simulink model "CSI_0313_SDC"  (R2019b)
settings: Solver=FixedStepDiscrete  StartTime=0.0  StopTime=Tstop  FixedStep=Tdelt  MaxStep=1e-4  RelTol=1e-3
values from neighbouring files (symbols this model uses):
  C = 12e-6    (= 1.2e-05)    [Inputparameter.m]
  Cdc = 4.76*10^-3    (= 0.00476)    [Inputparameter.m]
  Cemc = 1.5e-6    (= 1.5e-06)    [Inputparameter.m]
  enb = 0    [Run.m]
  fanalog = 7000    [Run.m]
  fTs = Update/18000    (= 0.000111111111111)    [Run.m]
  Ibase = 43*sqrt(2)    [Inputparameter.m]
  K120 = 0.0    (= 0)    [Run.m]
  K21 = 0.0    (= 0)    [Run.m]
  K5 = 0.0    (= 0)    [Run.m]
  K7 = 0.0    (= 0)    [Run.m]
  Kipll = 1.0    (= 1)    [Run.m]
  Klim = 1.03    [Run.m]
  Kpll = 20.0    (= 20)    [Run.m]
  Kpr = 0.9*Ibase/(Vbase)    [Run.m]
  Lgrid = 7.717e-4*10    (= 0.007717)    [Run.m]
  Lline = 60e-6    (= 6e-05)    [Inputparameter.m]
  Lpwm = 184.8e-6    (= 0.0001848)    [Inputparameter.m]
  mode = 1    [Run.m]
  Nsw = 18000/fbase    [Run.m]
  Qbpf = 1.0    (= 1)    [Run.m]
  Qpr = 1.0    (= 1)    [Run.m]
  Qs = 1    [Run.m]
  Rc = 10e-3    (= 0.01)    [Inputparameter.m]
  Remc = 1e-3    (= 0.001)    [Inputparameter.m]
  Rgrid = 2*pi*fbase*Lgrid/XR    [Run.m]
  Rline = 4.95e-3    (= 0.00495)    [Inputparameter.m]
  Rpre = 2.2    [Inputparameter.m]
  Rpwm = 6.2e-3    (= 0.0062)    [Inputparameter.m]
  Tdelt = (fTs)/(200*Update)    (= 2.77777777778e-07)    [Run.m]
  Tdt = 1.27e-6    (= 1.27e-06)    [Run.m]
  tstart = 0.2    [Run.m]
  Update = 2    [Run.m]
  Vbase = 400*sqrt(2/3)    [Inputparameter.m]
undefined symbols (not defined in the file or in its folder): sigbuilder_block
libraries: powerlib x54
(part 2 of 4)

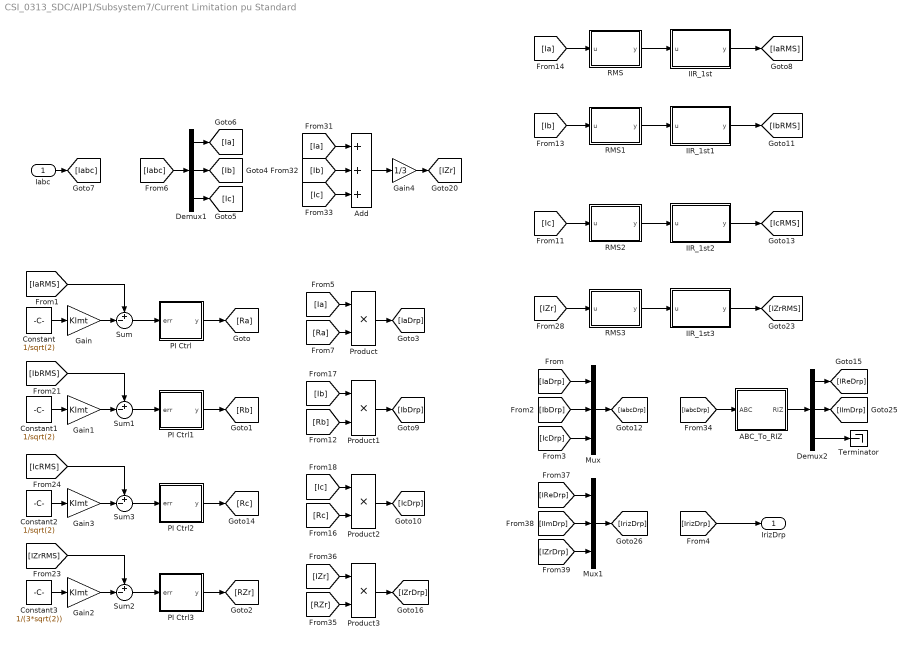
== system CSI_0313_SDC/AIP1/Subsystem7/Current Limitation pu Standard ==
  Iabc : Inport
  ABC_To_RIZ : MATLAB Function  TreatAsAtomicUnit=on
  Add : Sum  Inputs=+++
  Constant : Constant  Value=1/sqrt(2)
  Constant1 : Constant  Value=1/sqrt(2)
  Constant2 : Constant  Value=1/sqrt(2)
  Constant3 : Constant  Value=1/(3*sqrt(2))
  Demux1 : Demux  Outputs=3
  Demux2 : Demux  Outputs=3
  Gain{,1..3} (4 alike) : Gain  Gain=Klmt
  Gain4 : Gain  Gain=1/3
  IIR_1st : MATLAB Function  TreatAsAtomicUnit=on  mask{fc=100, fTs=fTs}
      mask prompts: fc "Cut-off frequency [Hz]"; fTs "Sample time [s]"
      mask help: 1st-order Low Pass Filter
  IIR_1st1 : MATLAB Function  TreatAsAtomicUnit=on  mask{fc=100, fTs=fTs}
      mask prompts: fc "Cut-off frequency [Hz]"; fTs "Sample time [s]"
      mask help: 1st-order Low Pass Filter
  IIR_1st2 : MATLAB Function  TreatAsAtomicUnit=on  mask{fc=100, fTs=fTs}
      mask prompts: fc "Cut-off frequency [Hz]"; fTs "Sample time [s]"
      mask help: 1st-order Low Pass Filter
  IIR_1st3 : MATLAB Function  TreatAsAtomicUnit=on  mask{fc=100, fTs=fTs}
      mask prompts: fc "Cut-off frequency [Hz]"; fTs "Sample time [s]"
      mask help: 1st-order Low Pass Filter
  Mux : Mux  Inputs=3
  Mux1 : Mux  Inputs=3
  PI Ctrl : MATLAB Function  TreatAsAtomicUnit=on  mask{fKP=0.005, fKI=100, fMinLmt=0, fMaxLmt=10, fTs=fTs}
      mask prompts: fKP "Proportional Gain"; fKI "Integral Coefficient"; fMinLmt "Minimum Limitation"; fMaxLmt "Maximum Limitation"; fTs "Sampling time [s]"
      mask help: Proportional Resonant Controller
  PI Ctrl1 : MATLAB Function  TreatAsAtomicUnit=on  mask{fKP=0.005, fKI=100, fMinLmt=0, fMaxLmt=10, fTs=fTs}
      mask prompts: fKP "Proportional Gain"; fKI "Integral Coefficient"; fMinLmt "Minimum Limitation"; fMaxLmt "Maximum Limitation"; fTs "Sampling time [s]"
      mask help: Proportional Resonant Controller
  PI Ctrl2 : MATLAB Function  TreatAsAtomicUnit=on  mask{fKP=0.005, fKI=100, fMinLmt=0, fMaxLmt=10, fTs=fTs}
      mask prompts: fKP "Proportional Gain"; fKI "Integral Coefficient"; fMinLmt "Minimum Limitation"; fMaxLmt "Maximum Limitation"; fTs "Sampling time [s]"
      mask help: Proportional Resonant Controller
  PI Ctrl3 : MATLAB Function  TreatAsAtomicUnit=on  mask{fKP=0.005, fKI=100, fMinLmt=0, fMaxLmt=10, fTs=fTs}
      mask prompts: fKP "Proportional Gain"; fKI "Integral Coefficient"; fMinLmt "Minimum Limitation"; fMaxLmt "Maximum Limitation"; fTs "Sampling time [s]"
      mask help: Proportional Resonant Controller
  Product{,1..3} (4 alike) : Product
  RMS : MATLAB Function  TreatAsAtomicUnit=on  mask{iNumAry=iRMSNum}
      mask prompts: iNumAry "RMS window points"
  RMS1 : MATLAB Function  TreatAsAtomicUnit=on  mask{iNumAry=iRMSNum}
      mask prompts: iNumAry "RMS window points"
  RMS2 : MATLAB Function  TreatAsAtomicUnit=on  mask{iNumAry=iRMSNum}
      mask prompts: iNumAry "RMS window points"
  RMS3 : MATLAB Function  TreatAsAtomicUnit=on  mask{iNumAry=iRMSNum}
      mask prompts: iNumAry "RMS window points"
  Sum{,1..3} (4 alike) : Sum  Inputs=+-|
  Terminator : Terminator
  IrizDrp : Outport
  wires:
  Demux2/3 -> Terminator/1
  Mux1/1 -> [IrizDrp]
  [IZrDrp] -> Mux1/3
  [IImDrp] -> Mux1/2
  [IReDrp] -> Mux1/1
  Demux2/2 -> [IImDrp]
  Demux2/1 -> [IReDrp]
  Product3/1 -> [IZrDrp]
  [RZr] -> Product3/2
  [IZr] -> Product3/1
  ABC_To_RIZ/1(RIZ) -> Demux2/1
  [IabcDrp] -> ABC_To_RIZ/1(ABC)
  Gain4/1 -> [IZr]
  [Ic] -> Add/3
  [Ib] -> Add/2
  [Ia] -> Add/1
  Add/1 -> Gain4/1
  Constant2/1 -> Gain3/1
  Sum3/1 -> PI Ctrl2/1(err)
  PI Ctrl2/1(y) -> [Rc]
  Gain3/1 -> Sum3/2
  [IcRMS] -> Sum3/1
  IIR_1st3/1(y) -> [IZrRMS]
  [IrizDrp] -> IrizDrp/1
  [IZr] -> RMS3/1(u)
  RMS3/1(y) -> IIR_1st3/1(u)
  Gain2/1 -> Sum2/2
  Constant3/1 -> Gain2/1
  Gain1/1 -> Sum1/2
  Constant1/1 -> Gain1/1
  Constant/1 -> Gain/1
  Gain/1 -> Sum/2
  IIR_1st2/1(y) -> [IcRMS]
  IIR_1st1/1(y) -> [IbRMS]
  IIR_1st/1(y) -> [IaRMS]
  RMS2/1(y) -> IIR_1st2/1(u)
  RMS1/1(y) -> IIR_1st1/1(u)
  RMS/1(y) -> IIR_1st/1(u)
  Sum2/1 -> PI Ctrl3/1(err)
  PI Ctrl3/1(y) -> [RZr]
  [IZrRMS] -> Sum2/1
  PI Ctrl1/1(y) -> [Rb]
  Sum1/1 -> PI Ctrl1/1(err)
  [IbRMS] -> Sum1/1
  Mux/1 -> [IabcDrp]
  Product2/1 -> [IcDrp]
  Product1/1 -> [IbDrp]
  Product/1 -> [IaDrp]
  [Rc] -> Product2/2
  [Ic] -> Product2/1
  [Rb] -> Product1/2
  [Ib] -> Product1/1
  [Ra] -> Product/2
  [Ia] -> Product/1
  Sum/1 -> PI Ctrl/1(err)
  [IcDrp] -> Mux/3
  [IbDrp] -> Mux/2
  [IaDrp] -> Mux/1
  PI Ctrl/1(y) -> [Ra]
  [IaRMS] -> Sum/1
  [Ib] -> RMS1/1(u)
  [Ic] -> RMS2/1(u)
  [Ia] -> RMS/1(u)
  Iabc/1 -> [Iabc]
  [Iabc] -> Demux1/1
  Demux1/1 -> [Ia]
  Demux1/3 -> [Ic]
  Demux1/2 -> [Ib]

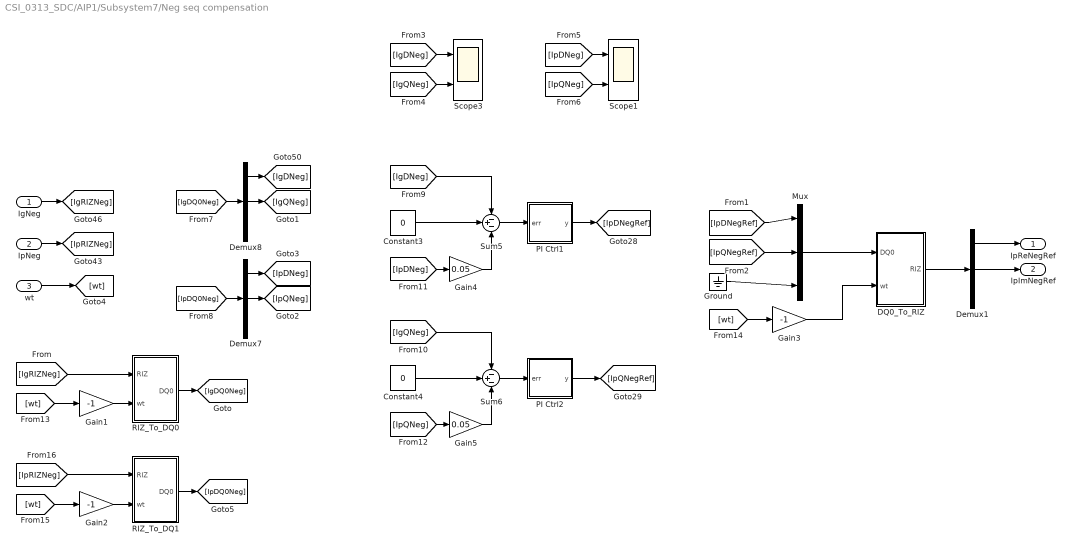
== system CSI_0313_SDC/AIP1/Subsystem7/Neg seq compensation ==
  IgNeg : Inport
  IpNeg : Inport  Port=2
  wt : Inport  Port=3
  Constant3 : Constant  Value=0  SampleTime=-1
  Constant4 : Constant  Value=0  SampleTime=-1
  DQ0_To_RIZ : MATLAB Function  TreatAsAtomicUnit=on  mask{iAxis=orient 90 degree behind A-axis}
      mask prompts: iAxis "Orient Axis Choice"
  Demux1 : Demux  Outputs=3
  Demux7 : Demux  Outputs=3
  Demux8 : Demux  Outputs=3
  Gain1 : Gain  Gain=-1
  Gain2 : Gain  Gain=-1
  Gain3 : Gain  Gain=-1
  Gain4 : Gain  Gain=0.05
  Gain5 : Gain  Gain=0.05
  Ground : Ground
  Mux : Mux  Inputs=3
  PI Ctrl1 : MATLAB Function  TreatAsAtomicUnit=on  mask{fKP=0.3, fKI=250, fMinLmt=-Ibase, fMaxLmt=Ibase, fTs=fTs}
      mask prompts: fKP "Proportional Gain"; fKI "Integral Coefficient"; fMinLmt "Minimum Limitation"; fMaxLmt "Maximum Limitation"; fTs "Sampling time [s]"
      mask help: Proportional Resonant Controller
  PI Ctrl2 : MATLAB Function  TreatAsAtomicUnit=on  mask{fKP=0.3, fKI=250, fMinLmt=-Ibase, fMaxLmt=Ibase, fTs=fTs}
      mask prompts: fKP "Proportional Gain"; fKI "Integral Coefficient"; fMinLmt "Minimum Limitation"; fMaxLmt "Maximum Limitation"; fTs "Sampling time [s]"
      mask help: Proportional Resonant Controller
  RIZ_To_DQ0 : MATLAB Function  TreatAsAtomicUnit=on  mask{iAxis=orient 90 degree behind A-axis}
      mask prompts: iAxis "Orient Axis Choice"
  RIZ_To_DQ1 : MATLAB Function  TreatAsAtomicUnit=on  mask{iAxis=orient 90 degree behind A-axis}
      mask prompts: iAxis "Orient Axis Choice"
  Scope1 : Scope  NumInputPorts=2
  Scope3 : Scope  NumInputPorts=2
  Sum5 : Sum  Inputs=-+-
  Sum6 : Sum  Inputs=-+-
  IpReNegRef : Outport  VectorParamsAs1DForOutWhenUnconnected=off
  IpImNegRef : Outport  Port=2  VectorParamsAs1DForOutWhenUnconnected=off
  wires:
  PI Ctrl1/1(y) -> [IpDNegRef]
  [IpQNeg] -> Gain5/1
  Demux8/2 -> [IgQNeg]
  Constant4/1 -> Sum6/2
  [IpDQ0Neg] -> Demux7/1
  Constant3/1 -> Sum5/2
  [IgDQ0Neg] -> Demux8/1
  Demux8/1 -> [IgDNeg]
  [IgDNeg] -> Sum5/1
  Demux7/2 -> [IpQNeg]
  [IpDNeg] -> Gain4/1
  [IgQNeg] -> Sum6/1
  Demux7/1 -> [IpDNeg]
  Sum5/1 -> PI Ctrl1/1(err)
  [IgDNeg] -> Scope3/1
  [IgQNeg] -> Scope3/2
  [IpDNeg] -> Scope1/1
  [IpQNeg] -> Scope1/2
  IgNeg/1 -> [IgRIZNeg]
  IpNeg/1 -> [IpRIZNeg]
  PI Ctrl2/1(y) -> [IpQNegRef]
  Sum6/1 -> PI Ctrl2/1(err)
  [IgRIZNeg] -> RIZ_To_DQ0/1(RIZ)
  wt/1 -> [wt]
  [wt] -> Gain1/1
  Gain1/1 -> RIZ_To_DQ0/2(wt)
  RIZ_To_DQ0/1(DQ0) -> [IgDQ0Neg]
  RIZ_To_DQ1/1(DQ0) -> [IpDQ0Neg]
  Gain2/1 -> RIZ_To_DQ1/2(wt)
  [wt] -> Gain2/1
  [IpRIZNeg] -> RIZ_To_DQ1/1(RIZ)
  [IpDNegRef] -> Mux/1
  [IpQNegRef] -> Mux/2
  Ground/1 -> Mux/3
  Mux/1 -> DQ0_To_RIZ/1(DQ0)
  [wt] -> Gain3/1
  Gain3/1 -> DQ0_To_RIZ/2(wt)
  DQ0_To_RIZ/1(RIZ) -> Demux1/1
  Demux1/1 -> IpReNegRef/1
  Demux1/2 -> IpImNegRef/1
  Gain4/1 -> Sum5/3
  Gain5/1 -> Sum6/3

== system CSI_0313_SDC/AIP1/Subsystem7/PLL ==
  Vabc : Inport
  ABC_To_RIZ : MATLAB Function  TreatAsAtomicUnit=on
  Constant : Constant  Value=2*pi*fFqBase  SampleTime=-1
  Constant1 : Constant  Value=2*pi
  Delay1 : Delay  DelayLength=1
  Delay2 : Delay  DelayLength=1
  Demux3 : Demux  Outputs=3
  Gain : Gain  Gain=1/(2*pi)
  Integral : MATLAB Function  TreatAsAtomicUnit=on  mask{fGain=1.0, fTs=fTs}
      mask prompts: fGain "Gain Value"; fTs "Sampling time [s]"
      mask help: Proportional Resonant Controller
  Math Function : Math  Operator=mod  SaturateOnIntegerOverflow=on
  PI Ctrl : MATLAB Function  TreatAsAtomicUnit=on  mask{fKP=fKPPLL, fKI=fKIPLL, fMinLmt=fDltMin, fMaxLmt=fDltMax, fTs=fTs}
      mask prompts: fKP "Proportional Gain"; fKI "Integral Coefficient"; fMinLmt "Minimum Limitation"; fMaxLmt "Maximum Limitation"; fTs "Sampling time [s]"
      mask help: Proportional Resonant Controller
  "Pos&Neg seq extract in subsystem " : Subsystem  mask{fQ=1.0, fTs=fTs}
      mask prompts: fQ "Quality Factor"; fTs "Sample Time"
  RIZ_To_DQ0 : MATLAB Function  TreatAsAtomicUnit=on  mask{iAxis=orient in A-axis}
      mask prompts: iAxis "Orient Axis Choice"
  Scope : Scope
  Sum : Sum  Inputs=++|
  Terminator : Terminator
  Terminator1 : Terminator
  f : Outport
  wt : Outport  Port=2
  VdPos : Outport  Port=3
  wires:
  Delay1/1 -> "Pos&Neg seq extract in subsystem "/2(ffc)
  "Pos&Neg seq extract in subsystem "/3(chk) -> [chk]
  [VdPos] -> VdPos/1
  [f] -> Delay1/1
  Demux3/3 -> Terminator1/1
  "Pos&Neg seq extract in subsystem "/2(RizNeg) -> Terminator/1
  "Pos&Neg seq extract in subsystem "/1(RizPos) -> [VrizPos]
  [Vriz] -> "Pos&Neg seq extract in subsystem "/1(RIZ)
  RIZ_To_DQ0/1(DQ0) -> Scope/1, [Vdq0Pos]
  [w] -> Gain/1
  [w] -> Integral/1(u)
  Gain/1 -> [f]
  Demux3/2 -> [VqPos]
  Demux3/1 -> [VdPos]
  [Vdq0Pos] -> Demux3/1
  PI Ctrl/1(y) -> Sum/2
  Sum/1 -> [w]
  [VrizPos] -> RIZ_To_DQ0/1(RIZ)
  Constant/1 -> Sum/1
  Vabc/1 -> [Vabc]
  Integral/1(y) -> Math Function/1
  Constant1/1 -> Math Function/2
  Math Function/1 -> [wt]
  [VqPos] -> PI Ctrl/1(err)
  [f] -> f/1
  [wt] -> Delay2/1
  Delay2/1 -> RIZ_To_DQ0/2(wt)
  [Vabc] -> ABC_To_RIZ/1(ABC)
  ABC_To_RIZ/1(RIZ) -> [Vriz]
  [wt] -> wt/1

== system CSI_0313_SDC/AIP1/Subsystem7/PR CSI Loop ==
  IrizRef : Inport
  Iriz : Inport  Port=2
  IrizDrp : Inport  Port=3
  fPLL : Inport  Port=4
  Demux1 : Demux  Outputs=3
  Demux2 : Demux  Outputs=3
  Demux3 : Demux  Outputs=3
  Mux3 : Mux  Inputs=3
  PR Ctrl : MATLAB Function  TreatAsAtomicUnit=on  mask{fP=fKP, fQ=fKQ, fTs=fTs}
      mask prompts: fP "Proportional Gain"; fQ "Quality Factor"; fTs "Sampling time [s]"
      mask help: Proportional Resonant Controller
  PR Ctrl1 : MATLAB Function  TreatAsAtomicUnit=on  mask{fP=fKP, fQ=fKQ, fTs=fTs}
      mask prompts: fP "Proportional Gain"; fQ "Quality Factor"; fTs "Sampling time [s]"
      mask help: Proportional Resonant Controller
  PR Ctrl2 : MATLAB Function  TreatAsAtomicUnit=on  mask{fP=fKP*mode, fQ=fKQ, fTs=fTs}
      mask prompts: fP "Proportional Gain"; fQ "Quality Factor"; fTs "Sampling time [s]"
      mask help: Proportional Resonant Controller
  RIZ_To_ABC : MATLAB Function  TreatAsAtomicUnit=on
  Sum : Sum  Inputs=-+-
  Sum1 : Sum  Inputs=-+-
  Sum2 : Sum  Inputs=-+-
  VabcFB : Outport
  wires:
  Sum2/1 -> PR Ctrl2/1(err)
  Sum1/1 -> PR Ctrl1/1(err)
  Sum/1 -> PR Ctrl/1(err)
  [VabcFB] -> VabcFB/1
  fPLL/1 -> [fPLL]
  IrizDrp/1 -> [IrizDrp]
  [IrizDrp] -> Demux2/1
  Demux2/3 -> [IZrDrp]
  Demux2/1 -> [IReDrp]
  Demux2/2 -> [IImDrp]
  Demux1/2 -> [IImRef]
  [IrizRef] -> Demux1/1
  Demux1/1 -> [IReRef]
  Demux1/3 -> [IZrRef]
  IrizRef/1 -> [IrizRef]
  Iriz/1 -> [Iriz]
  Demux3/3 -> [IZr]
  Demux3/1 -> [IRe]
  Demux3/2 -> [IIm]
  [Iriz] -> Demux3/1
  PR Ctrl2/1(y) -> [VZrFB]
  [IImDrp] -> Sum1/3
  [IZr] -> Sum2/1
  Mux3/1 -> RIZ_To_ABC/1(RIZ)
  [fPLL] -> PR Ctrl1/2(ffc)
  RIZ_To_ABC/1(ABC) -> [VabcFB]
  [IReDrp] -> Sum/3
  [fPLL] -> PR Ctrl/2(ffc)
  [IIm] -> Sum1/1
  [fPLL] -> PR Ctrl2/2(ffc)
  [IImRef] -> Sum1/2
  [VReFB] -> Mux3/1
  [VZrFB] -> Mux3/3
  [IRe] -> Sum/1
  PR Ctrl1/1(y) -> [VImFB]
  PR Ctrl/1(y) -> [VReFB]
  [IZrRef] -> Sum2/2
  [IZrDrp] -> Sum2/3
  [IReRef] -> Sum/2
  [VImFB] -> Mux3/2

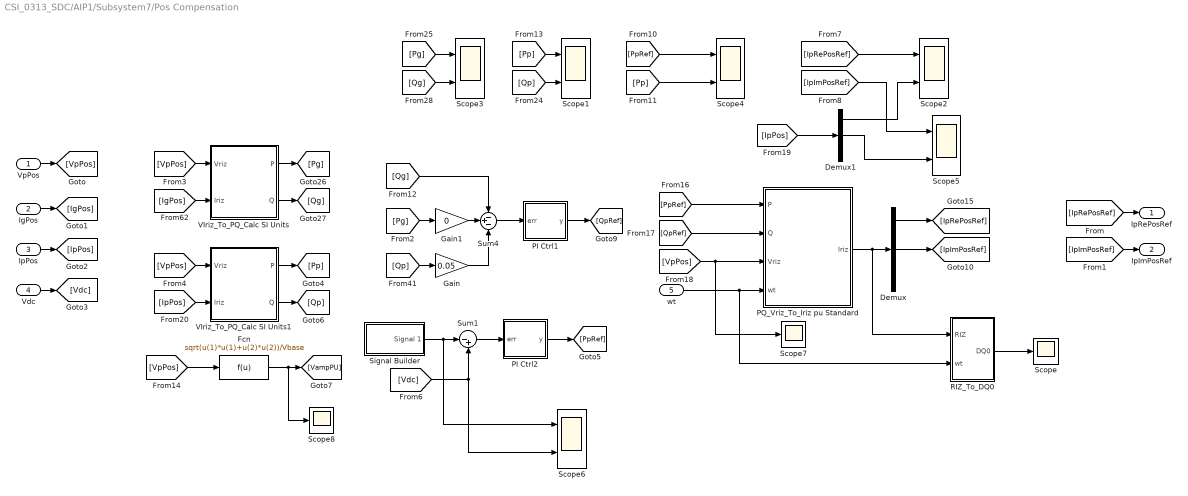
== system CSI_0313_SDC/AIP1/Subsystem7/Pos Compensation ==
  VpPos : Inport
  IgPos : Inport  Port=2
  IpPos : Inport  Port=3
  Vdc : Inport  Port=4
  wt : Inport  Port=5
  Demux : Demux  Outputs=3
  Demux1 : Demux  Outputs=3
  Fcn : Fcn  Expr=sqrt(u(1)*u(1)+u(2)*u(2))/Vbase
  Gain : Gain  Gain=0.05
  Gain1 : Gain  Gain=0
  PI Ctrl1 : MATLAB Function  TreatAsAtomicUnit=on  mask{fKP=0.3, fKI=200, fMinLmt=-30, fMaxLmt=30, fTs=fTs}
      mask prompts: fKP "Proportional Gain"; fKI "Integral Coefficient"; fMinLmt "Minimum Limitation"; fMaxLmt "Maximum Limitation"; fTs "Sampling time [s]"
      mask help: Proportional Resonant Controller
  PI Ctrl2 : MATLAB Function  TreatAsAtomicUnit=on  mask{fKP=0.05, fKI=0, fMinLmt=-30, fMaxLmt=30, fTs=fTs}
      mask prompts: fKP "Proportional Gain"; fKI "Integral Coefficient"; fMinLmt "Minimum Limitation"; fMaxLmt "Maximum Limitation"; fTs "Sampling time [s]"
      mask help: Proportional Resonant Controller
  PQ_Vriz_To_Iriz pu Standard : MATLAB Function  TreatAsAtomicUnit=on  mask{Ibase=Ibase}
      mask prompts: Ibase "Current base"
  RIZ_To_DQ0 : MATLAB Function  TreatAsAtomicUnit=on  mask{iAxis=orient 90 degree behind A-axis}
      mask prompts: iAxis "Orient Axis Choice"
  Scope : Scope
  Scope{1..6} (6 alike) : Scope  NumInputPorts=2
  Scope7 : Scope
  Scope8 : Scope
  Signal Builder : Subsystem  Tag=STV Subsys  LoadFcn=sigbuilder_block('load');  StartFcn=sigbuilder_block('start');  StopFcn=sigbuilder_block('stop');  ClipboardFcn=sigbuilder_block('clipboard');  mask(Sigbuilder block){tuvar=[0:10]}
      mask help: Simulink:masks:SigbuilderBlock_MD
      mask init:
      | if ~strcmp(get_param(bdroot(gcbh),'SimulationStatus'),'stopped') tuvar = sigbuilder_block('maskInit'); end
      settings: CopyFcn=sigbuilder_block('copy');  DeleteFcn=sigbuilder_block('delete');  ModelCloseFcn=sigbuilder_block('modelClose');  PreSaveFcn=sigbuilder_block('preSave');  PauseFcn=sigbuilder_block('pause');  ContinueFcn=sigbuilder_block('continue');  NameChangeFcn=sigbuilder_block('namechange');  OpenFcn=sigbuilder_block('open',[403.2 79.8 550.8 400.2 ]);  CloseFcn=sigbuilder_block('close');
      mask Display: plot(0, 0, 100, 100,[2, 2, 32, 32, 2], [68, 8, 8, 68, 68],[32, 2], [38, 38], [32, 19, 2],[53, 60, 44], [32, 17, 17, 2],[16, 16, 31, 31]);txt = getActiveGroup(gcbh);text(2, 100, txt,'verticalAlignment', 'top');
  Sum1 : Sum  Inputs=|-+
  Sum4 : Sum  Inputs=-+-
  VIriz_To_PQ_Calc SI Units : MATLAB Function  TreatAsAtomicUnit=on
  VIriz_To_PQ_Calc SI Units1 : MATLAB Function  TreatAsAtomicUnit=on
  IpRePosRef : Outport  VectorParamsAs1DForOutWhenUnconnected=off
  IpImPosRef : Outport  Port=2  VectorParamsAs1DForOutWhenUnconnected=off
  wires:
  [VpPos] -> VIriz_To_PQ_Calc SI Units/1(Vriz)
  VIriz_To_PQ_Calc SI Units/2(Q) -> [Qg]
  [IpPos] -> VIriz_To_PQ_Calc SI Units1/2(Iriz)
  VIriz_To_PQ_Calc SI Units1/2(Q) -> [Qp]
  [IgPos] -> VIriz_To_PQ_Calc SI Units/2(Iriz)
  [Qp] -> Gain/1
  VIriz_To_PQ_Calc SI Units1/1(P) -> [Pp]
  Sum4/1 -> PI Ctrl1/1(err)
  [VpPos] -> VIriz_To_PQ_Calc SI Units1/1(Vriz)
  VIriz_To_PQ_Calc SI Units/1(P) -> [Pg]
  PI Ctrl1/1(y) -> [QpRef]
  Gain/1 -> Sum4/3
  [Qg] -> Scope3/2
  [Qg] -> Sum4/1
  [Pg] -> Scope3/1
  Demux/1 -> [IpRePosRef]
  [Pp] -> Scope1/1
  Demux/2 -> [IpImPosRef]
  VpPos/1 -> [VpPos]
  IgPos/1 -> [IgPos]
  IpPos/1 -> [IpPos]
  [IpRePosRef] -> IpRePosRef/1
  [IpImPosRef] -> IpImPosRef/1
  [Qp] -> Scope1/2
  [Pg] -> Gain1/1
  Gain1/1 -> Sum4/2
  Vdc/1 -> [Vdc]
  Sum1/1 -> PI Ctrl2/1(err)
  PI Ctrl2/1(y) -> [PpRef]
  [PpRef] -> Scope4/1
  [Pp] -> Scope4/2
  wt/1 -> RIZ_To_DQ0/2(wt), PQ_Vriz_To_Iriz pu Standard/4(wt)
  [VpPos] -> Fcn/1
  Fcn/1 -> Scope8/1, [VampPU]
  [PpRef] -> PQ_Vriz_To_Iriz pu Standard/1(P)
  [QpRef] -> PQ_Vriz_To_Iriz pu Standard/2(Q)
  [IpPos] -> Demux1/1
  [IpRePosRef] -> Scope2/1
  Demux1/1 -> Scope2/2
  [IpImPosRef] -> Scope5/1
  Demux1/2 -> Scope5/2
  PQ_Vriz_To_Iriz pu Standard/1(Iriz) -> RIZ_To_DQ0/1(RIZ), Demux/1
  [Vdc] -> Scope6/2, Sum1/2
  Signal Builder/1(Signal 1) -> Scope6/1, Sum1/1
  RIZ_To_DQ0/1(DQ0) -> Scope/1
  [VpPos] -> PQ_Vriz_To_Iriz pu Standard/3(Vriz), Scope7/1

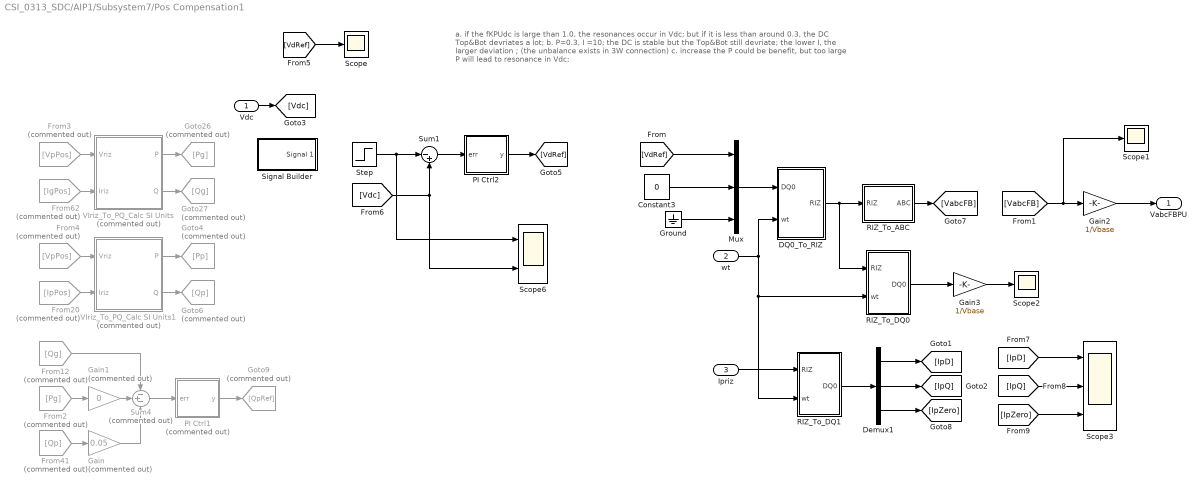
== system CSI_0313_SDC/AIP1/Subsystem7/Pos Compensation1 ==
  note: a. if the fKPUdc is large than 1.0, the resonances occur in Vdc; but if it is less than around 0.3, the DC Top&Bot devriates a lot;
      | b. P=0.3, I =10; the DC is stable but the Top&Bot still devriate; the lower I, the larger deviation；(the unbalance exists in 3W connection)
      | c. increase the P could be benefit, but too large P will lead to resonance in Vdc;
  Vdc : Inport
  wt : Inport  Port=2
  Ipriz : Inport  Port=3
  Constant3 : Constant  Value=0  SampleTime=-1
  DQ0_To_RIZ : MATLAB Function  TreatAsAtomicUnit=on  mask{iAxis=orient in A-axis}
      mask prompts: iAxis "Orient Axis Choice"
  Demux1 : Demux  Outputs=3
  From12 : From  Commented=on  GotoTag=Qg
  From2 : From  Commented=on  GotoTag=Pg
  From20 : From  Commented=on  GotoTag=IpPos
  From3 : From  Commented=on  GotoTag=VpPos
  From4 : From  Commented=on  GotoTag=VpPos
  From41 : From  Commented=on  GotoTag=Qp
  From62 : From  Commented=on  GotoTag=IgPos
  Gain : Gain  Commented=on  Gain=0.05
  Gain1 : Gain  Commented=on  Gain=0
  Gain2 : Gain  Gain=1/Vbase
  Gain3 : Gain  Gain=1/Vbase
  Goto26 : Goto  Commented=on  GotoTag=Pg
  Goto27 : Goto  Commented=on  GotoTag=Qg
  Goto4 : Goto  Commented=on  GotoTag=Pp
  Goto6 : Goto  Commented=on  GotoTag=Qp
  Goto9 : Goto  Commented=on  GotoTag=QpRef
  Ground : Ground
  Mux : Mux  Inputs=3
  PI Ctrl1 : MATLAB Function  Commented=on  TreatAsAtomicUnit=on  mask{fKP=0.3, fKI=200, fMinLmt=-30, fMaxLmt=30, fTs=fTs}
      mask prompts: fKP "Proportional Gain"; fKI "Integral Coefficient"; fMinLmt "Minimum Limitation"; fMaxLmt "Maximum Limitation"; fTs "Sampling time [s]"
      mask help: Proportional Resonant Controller
  PI Ctrl2 : MATLAB Function  TreatAsAtomicUnit=on  mask{fKP=0.4, fKI=6, fMinLmt=-0.3*Vbase, fMaxLmt=0.3*Vbase, fTs=fTs}
      mask prompts: fKP "Proportional Gain"; fKI "Integral Coefficient"; fMinLmt "Minimum Limitation"; fMaxLmt "Maximum Limitation"; fTs "Sampling time [s]"
      mask help: Proportional Resonant Controller
  RIZ_To_ABC : MATLAB Function  TreatAsAtomicUnit=on
  RIZ_To_DQ0 : MATLAB Function  TreatAsAtomicUnit=on  mask{iAxis=orient in A-axis}
      mask prompts: iAxis "Orient Axis Choice"
  RIZ_To_DQ1 : MATLAB Function  TreatAsAtomicUnit=on  mask{iAxis=orient in A-axis}
      mask prompts: iAxis "Orient Axis Choice"
  Scope : Scope
  Scope1 : Scope
  Scope2 : Scope
  Scope3 : Scope  NumInputPorts=3
  Scope6 : Scope  NumInputPorts=2
  Signal Builder : Subsystem  Tag=STV Subsys  LoadFcn=sigbuilder_block('load');  StartFcn=sigbuilder_block('start');  StopFcn=sigbuilder_block('stop');  ClipboardFcn=sigbuilder_block('clipboard');  mask(Sigbuilder block){tuvar=[0:10]}
      mask help: Simulink:masks:SigbuilderBlock_MD
      mask init:
      | if ~strcmp(get_param(bdroot(gcbh),'SimulationStatus'),'stopped') tuvar = sigbuilder_block('maskInit'); end
      settings: CopyFcn=sigbuilder_block('copy');  DeleteFcn=sigbuilder_block('delete');  ModelCloseFcn=sigbuilder_block('modelClose');  PreSaveFcn=sigbuilder_block('preSave');  PauseFcn=sigbuilder_block('pause');  ContinueFcn=sigbuilder_block('continue');  NameChangeFcn=sigbuilder_block('namechange');  OpenFcn=sigbuilder_block('open',[403.2 79.8 550.8 400.2 ]);  CloseFcn=sigbuilder_block('close');
      mask Display: plot(0, 0, 100, 100,[2, 2, 32, 32, 2], [68, 8, 8, 68, 68],[32, 2], [38, 38], [32, 19, 2],[53, 60, 44], [32, 17, 17, 2],[16, 16, 31, 31]);txt = getActiveGroup(gcbh);text(2, 100, txt,'verticalAlignment', 'top');
  Step : Step  Time=0.5  Before=650  After=700
  Sum1 : Sum  Inputs=|-+
  Sum4 : Sum  Commented=on  Inputs=-+-
  VIriz_To_PQ_Calc SI Units : MATLAB Function  Commented=on  TreatAsAtomicUnit=on
  VIriz_To_PQ_Calc SI Units1 : MATLAB Function  Commented=on  TreatAsAtomicUnit=on
  VabcFBPU : Outport  VectorParamsAs1DForOutWhenUnconnected=off
  wires:
  [Vdc] -> Sum1/2, Scope6/2
  PI Ctrl2/1(y) -> [VdRef]
  Sum1/1 -> PI Ctrl2/1(err)
  Vdc/1 -> [Vdc]
  Gain1/1 -> Sum4/2
  From2/1 -> Gain1/1
  [VabcFB] -> Scope1/1, Gain2/1
  [VdRef] -> Scope/1
  From12/1 -> Sum4/1
  Gain/1 -> Sum4/3
  PI Ctrl1/1(y) -> Goto9/1
  VIriz_To_PQ_Calc SI Units/1(P) -> Goto26/1
  From4/1 -> VIriz_To_PQ_Calc SI Units1/1(Vriz)
  Sum4/1 -> PI Ctrl1/1(err)
  VIriz_To_PQ_Calc SI Units1/1(P) -> Goto4/1
  From41/1 -> Gain/1
  From62/1 -> VIriz_To_PQ_Calc SI Units/2(Iriz)
  VIriz_To_PQ_Calc SI Units1/2(Q) -> Goto6/1
  From20/1 -> VIriz_To_PQ_Calc SI Units1/2(Iriz)
  VIriz_To_PQ_Calc SI Units/2(Q) -> Goto27/1
  From3/1 -> VIriz_To_PQ_Calc SI Units/1(Vriz)
  Ground/1 -> Mux/3
  Mux/1 -> DQ0_To_RIZ/1(DQ0)
  wt/1 -> RIZ_To_DQ0/2(wt), RIZ_To_DQ1/2(wt), DQ0_To_RIZ/2(wt)
  RIZ_To_ABC/1(ABC) -> [VabcFB]
  DQ0_To_RIZ/1(RIZ) -> RIZ_To_DQ0/1(RIZ), RIZ_To_ABC/1(RIZ)
  Gain2/1 -> VabcFBPU/1
  RIZ_To_DQ0/1(DQ0) -> Gain3/1
  Gain3/1 -> Scope2/1
  Step/1 -> Scope6/1, Sum1/1
  [VdRef] -> Mux/1
  Ipriz/1 -> RIZ_To_DQ1/1(RIZ)
  RIZ_To_DQ1/1(DQ0) -> Demux1/1
  Demux1/1 -> [IpD]
  Demux1/2 -> [IpQ]
  Constant3/1 -> Mux/2
  [IpD] -> Scope3/1
  [IpQ] -> Scope3/2
  Demux1/3 -> [IpZero]
  [IpZero] -> Scope3/3

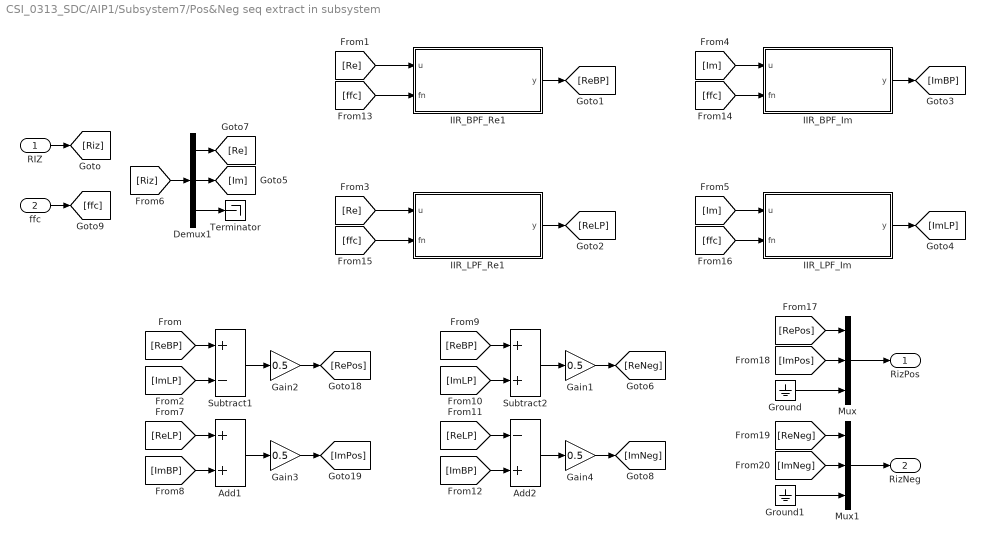
== system CSI_0313_SDC/AIP1/Subsystem7/Pos&Neg seq extract in subsystem  ==
  RIZ : Inport
  ffc : Inport  Port=2
  Add1 : Sum
  Add2 : Sum  Inputs=-+
  Demux1 : Demux  Outputs=3
  Gain{1..4} (4 alike) : Gain  Gain=0.5
  Ground : Ground
  Ground1 : Ground
  IIR_BPF_Im : MATLAB Function  TreatAsAtomicUnit=on  mask{fQ=fQ, fTs=fTs, iMode=IIR2 used as BPF in SOGI}
      mask prompts: fQ "Quality factor"; fTs "Sample time [s]"; iMode "Modes of 2nd-order transfer function"
  IIR_BPF_Re1 : MATLAB Function  TreatAsAtomicUnit=on  mask{fQ=fQ, fTs=fTs, iMode=IIR2 used as BPF in SOGI}
      mask prompts: fQ "Quality factor"; fTs "Sample time [s]"; iMode "Modes of 2nd-order transfer function"
  IIR_LPF_Im : MATLAB Function  TreatAsAtomicUnit=on  mask{fQ=fQ, fTs=fTs, iMode=IIR2 used as LPF in SOGI}
      mask prompts: fQ "Quality factor"; fTs "Sample time [s]"; iMode "Modes of 2nd-order transfer function"
  IIR_LPF_Re1 : MATLAB Function  TreatAsAtomicUnit=on  mask{fQ=fQ, fTs=fTs, iMode=IIR2 used as LPF in SOGI}
      mask prompts: fQ "Quality factor"; fTs "Sample time [s]"; iMode "Modes of 2nd-order transfer function"
  Mux : Mux  Inputs=3
  Mux1 : Mux  Inputs=3
  Subtract1 : Sum  Inputs=+-
  Subtract2 : Sum
  Terminator : Terminator
  RizPos : Outport
  RizNeg : Outport  Port=2
  wires:
  [ImBP] -> Add2/2
  [ffc] -> IIR_BPF_Im/2(fn)
  Add1/1 -> Gain3/1
  Demux1/1 -> [Re]
  RIZ/1 -> [Riz]
  Ground1/1 -> Mux1/3
  Add2/1 -> Gain4/1
  [ImLP] -> Subtract1/2
  [ReLP] -> Add1/1
  [ReBP] -> Subtract2/1
  [ImBP] -> Add1/2
  Gain1/1 -> [ReNeg]
  IIR_LPF_Re1/1(y) -> [ReLP]
  [Re] -> IIR_BPF_Re1/1(u)
  [RePos] -> Mux/1
  [ReBP] -> Subtract1/1
  Mux/1 -> RizPos/1
  [ffc] -> IIR_BPF_Re1/2(fn)
  Mux1/1 -> RizNeg/1
  IIR_BPF_Im/1(y) -> [ImBP]
  [Im] -> IIR_BPF_Im/1(u)
  Demux1/3 -> Terminator/1
  IIR_BPF_Re1/1(y) -> [ReBP]
  Gain3/1 -> [ImPos]
  IIR_LPF_Im/1(y) -> [ImLP]
  [ImNeg] -> Mux1/2
  [Im] -> IIR_LPF_Im/1(u)
  [ffc] -> IIR_LPF_Im/2(fn)
  [ImLP] -> Subtract2/2
  Demux1/2 -> [Im]
  Subtract1/1 -> Gain2/1
  [Re] -> IIR_LPF_Re1/1(u)
  [ffc] -> IIR_LPF_Re1/2(fn)
  [Riz] -> Demux1/1
  Ground/1 -> Mux/3
  [ReNeg] -> Mux1/1
  Gain4/1 -> [ImNeg]
  Subtract2/1 -> Gain1/1
  Gain2/1 -> [RePos]
  [ReLP] -> Add2/1
  ffc/1 -> [ffc]
  [ImPos] -> Mux/2

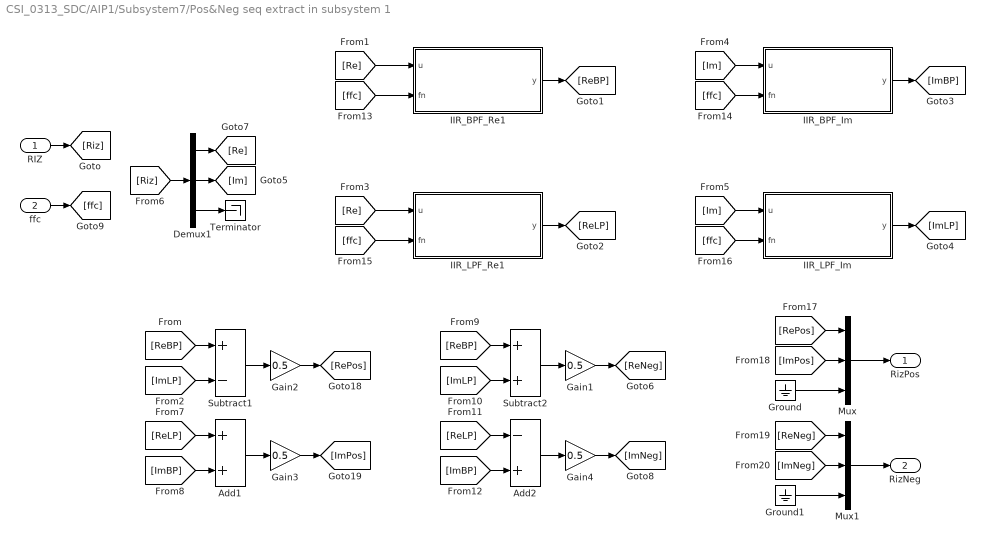
== system CSI_0313_SDC/AIP1/Subsystem7/Pos&Neg seq extract in subsystem 1 ==
  RIZ : Inport
  ffc : Inport  Port=2
  Add1 : Sum
  Add2 : Sum  Inputs=-+
  Demux1 : Demux  Outputs=3
  Gain{1..4} (4 alike) : Gain  Gain=0.5
  Ground : Ground
  Ground1 : Ground
  IIR_BPF_Im : MATLAB Function  TreatAsAtomicUnit=on  mask{fQ=fQ, fTs=fTs, iMode=IIR2 used as BPF in SOGI}
      mask prompts: fQ "Quality factor"; fTs "Sample time [s]"; iMode "Modes of 2nd-order transfer function"
  IIR_BPF_Re1 : MATLAB Function  TreatAsAtomicUnit=on  mask{fQ=fQ, fTs=fTs, iMode=IIR2 used as BPF in SOGI}
      mask prompts: fQ "Quality factor"; fTs "Sample time [s]"; iMode "Modes of 2nd-order transfer function"
  IIR_LPF_Im : MATLAB Function  TreatAsAtomicUnit=on  mask{fQ=fQ, fTs=fTs, iMode=IIR2 used as LPF in SOGI}
      mask prompts: fQ "Quality factor"; fTs "Sample time [s]"; iMode "Modes of 2nd-order transfer function"
  IIR_LPF_Re1 : MATLAB Function  TreatAsAtomicUnit=on  mask{fQ=fQ, fTs=fTs, iMode=IIR2 used as LPF in SOGI}
      mask prompts: fQ "Quality factor"; fTs "Sample time [s]"; iMode "Modes of 2nd-order transfer function"
  Mux : Mux  Inputs=3
  Mux1 : Mux  Inputs=3
  Subtract1 : Sum  Inputs=+-
  Subtract2 : Sum
  Terminator : Terminator
  RizPos : Outport
  RizNeg : Outport  Port=2
  wires:
  [ImPos] -> Mux/2
  ffc/1 -> [ffc]
  [ReLP] -> Add2/1
  Gain2/1 -> [RePos]
  Subtract2/1 -> Gain1/1
  Gain4/1 -> [ImNeg]
  [ReNeg] -> Mux1/1
  Ground/1 -> Mux/3
  [Riz] -> Demux1/1
  [ffc] -> IIR_LPF_Re1/2(fn)
  [Re] -> IIR_LPF_Re1/1(u)
  Subtract1/1 -> Gain2/1
  Demux1/2 -> [Im]
  [ImLP] -> Subtract2/2
  [ffc] -> IIR_LPF_Im/2(fn)
  [Im] -> IIR_LPF_Im/1(u)
  [ImNeg] -> Mux1/2
  IIR_LPF_Im/1(y) -> [ImLP]
  Gain3/1 -> [ImPos]
  IIR_BPF_Re1/1(y) -> [ReBP]
  Demux1/3 -> Terminator/1
  [Im] -> IIR_BPF_Im/1(u)
  IIR_BPF_Im/1(y) -> [ImBP]
  Mux1/1 -> RizNeg/1
  [ffc] -> IIR_BPF_Re1/2(fn)
  Mux/1 -> RizPos/1
  [ReBP] -> Subtract1/1
  [RePos] -> Mux/1
  [Re] -> IIR_BPF_Re1/1(u)
  IIR_LPF_Re1/1(y) -> [ReLP]
  Gain1/1 -> [ReNeg]
  [ImBP] -> Add1/2
  [ReBP] -> Subtract2/1
  [ReLP] -> Add1/1
  [ImLP] -> Subtract1/2
  Add2/1 -> Gain4/1
  Ground1/1 -> Mux1/3
  RIZ/1 -> [Riz]
  Demux1/1 -> [Re]
  Add1/1 -> Gain3/1
  [ffc] -> IIR_BPF_Im/2(fn)
  [ImBP] -> Add2/2

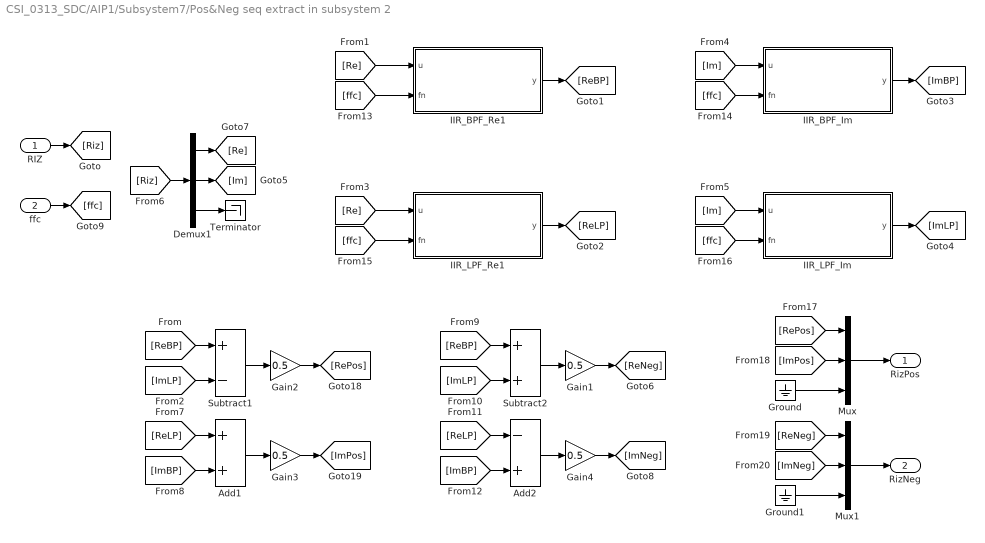
== system CSI_0313_SDC/AIP1/Subsystem7/Pos&Neg seq extract in subsystem 2 ==
  RIZ : Inport
  ffc : Inport  Port=2
  Add1 : Sum
  Add2 : Sum  Inputs=-+
  Demux1 : Demux  Outputs=3
  Gain{1..4} (4 alike) : Gain  Gain=0.5
  Ground : Ground
  Ground1 : Ground
  IIR_BPF_Im : MATLAB Function  TreatAsAtomicUnit=on  mask{fQ=fQ, fTs=fTs, iMode=IIR2 used as BPF in SOGI}
      mask prompts: fQ "Quality factor"; fTs "Sample time [s]"; iMode "Modes of 2nd-order transfer function"
  IIR_BPF_Re1 : MATLAB Function  TreatAsAtomicUnit=on  mask{fQ=fQ, fTs=fTs, iMode=IIR2 used as BPF in SOGI}
      mask prompts: fQ "Quality factor"; fTs "Sample time [s]"; iMode "Modes of 2nd-order transfer function"
  IIR_LPF_Im : MATLAB Function  TreatAsAtomicUnit=on  mask{fQ=fQ, fTs=fTs, iMode=IIR2 used as LPF in SOGI}
      mask prompts: fQ "Quality factor"; fTs "Sample time [s]"; iMode "Modes of 2nd-order transfer function"
  IIR_LPF_Re1 : MATLAB Function  TreatAsAtomicUnit=on  mask{fQ=fQ, fTs=fTs, iMode=IIR2 used as LPF in SOGI}
      mask prompts: fQ "Quality factor"; fTs "Sample time [s]"; iMode "Modes of 2nd-order transfer function"
  Mux : Mux  Inputs=3
  Mux1 : Mux  Inputs=3
  Subtract1 : Sum  Inputs=+-
  Subtract2 : Sum
  Terminator : Terminator
  RizPos : Outport
  RizNeg : Outport  Port=2
  wires:
  [ImBP] -> Add2/2
  [ffc] -> IIR_BPF_Im/2(fn)
  Add1/1 -> Gain3/1
  Demux1/1 -> [Re]
  RIZ/1 -> [Riz]
  Ground1/1 -> Mux1/3
  Add2/1 -> Gain4/1
  [ImLP] -> Subtract1/2
  [ReLP] -> Add1/1
  [ReBP] -> Subtract2/1
  [ImBP] -> Add1/2
  Gain1/1 -> [ReNeg]
  IIR_LPF_Re1/1(y) -> [ReLP]
  [Re] -> IIR_BPF_Re1/1(u)
  [RePos] -> Mux/1
  [ReBP] -> Subtract1/1
  Mux/1 -> RizPos/1
  [ffc] -> IIR_BPF_Re1/2(fn)
  Mux1/1 -> RizNeg/1
  IIR_BPF_Im/1(y) -> [ImBP]
  [Im] -> IIR_BPF_Im/1(u)
  Demux1/3 -> Terminator/1
  IIR_BPF_Re1/1(y) -> [ReBP]
  Gain3/1 -> [ImPos]
  IIR_LPF_Im/1(y) -> [ImLP]
  [ImNeg] -> Mux1/2
  [Im] -> IIR_LPF_Im/1(u)
  [ffc] -> IIR_LPF_Im/2(fn)
  [ImLP] -> Subtract2/2
  Demux1/2 -> [Im]
  Subtract1/1 -> Gain2/1
  [Re] -> IIR_LPF_Re1/1(u)
  [ffc] -> IIR_LPF_Re1/2(fn)
  [Riz] -> Demux1/1
  Ground/1 -> Mux/3
  [ReNeg] -> Mux1/1
  Gain4/1 -> [ImNeg]
  Subtract2/1 -> Gain1/1
  Gain2/1 -> [RePos]
  [ReLP] -> Add2/1
  ffc/1 -> [ffc]
  [ImPos] -> Mux/2

== system CSI_0313_SDC/AIP1/Subsystem7/Subsystem5 ==
  Vabc : Inport
  Vdc : Inport  Port=2
  3rd Injection1 : MATLAB Function  TreatAsAtomicUnit=on  mask{mode=mode}
      mask prompts: mode "Three wire/four wire"
  Vmod : Outport
  wires:
  Vabc/1 -> 3rd Injection1/1(Vabc)
  3rd Injection1/1(Mod) -> Vmod/1
  Vdc/1 -> 3rd Injection1/2(Vdc)

== system CSI_0313_SDC/AIP1/Subsystem7/Zero seq compensation ==
  IgRIZ : Inport
  IpRIZ : Inport  Port=2
  IrizLmtPU : Inport  Port=3
  Freq : Inport  Port=4
  Demux1 : Demux  Outputs=3
  Demux2 : Demux  Outputs=3
  Demux3 : Demux  Outputs=3
  Gain1 : Gain  Gain=Ibase
  Gain5 : Gain  Gain=0.05
  PR Ctrl1 : MATLAB Function  TreatAsAtomicUnit=on  mask{fP=0.4, fQ=1.0, fTs=fTs}
      mask prompts: fP "Proportional Gain"; fQ "Quality Factor"; fTs "Sampling time [s]"
      mask help: Proportional Resonant Controller
  Scope3 : Scope  NumInputPorts=2
  Sum7 : Sum  Inputs=---
  IpZrRef : Outport  VectorParamsAs1DForOutWhenUnconnected=off
  wires:
  [IgZr] -> Sum7/1
  PR Ctrl1/1(y) -> [IpZrRef]
  Sum7/1 -> PR Ctrl1/1(err)
  Demux3/3 -> Gain1/1
  IrizLmtPU/1 -> Demux3/1
  Demux1/3 -> [IpZr]
  IpRIZ/1 -> Demux1/1
  [IpZrRef] -> IpZrRef/1
  Demux2/3 -> [IgZr]
  IgRIZ/1 -> Demux2/1
  [IgZr] -> Scope3/1
  [IpZr] -> Scope3/2
  Gain5/1 -> Sum7/2
  [IpZr] -> Gain5/1
  Freq/1 -> PR Ctrl1/2(ffc)
  Gain1/1 -> [IzrLmtDrp]
  [IzrLmtDrp] -> Sum7/3

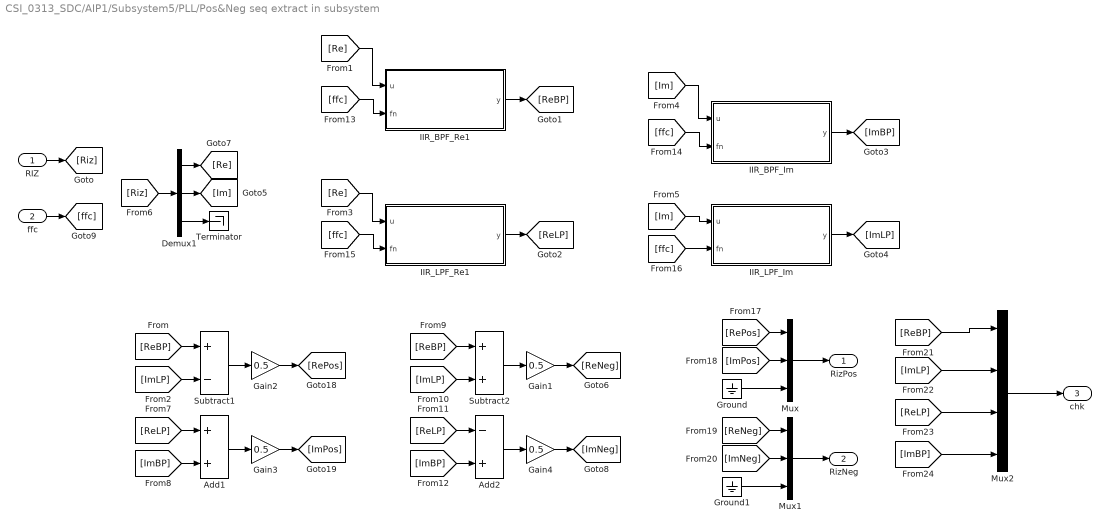
== system CSI_0313_SDC/AIP1/Subsystem5/PLL/Pos&Neg seq extract in subsystem  ==
  RIZ : Inport
  ffc : Inport  Port=2
  Add1 : Sum
  Add2 : Sum  Inputs=-+
  Demux1 : Demux  Outputs=3
  Gain{1..4} (4 alike) : Gain  Gain=0.5
  Ground : Ground
  Ground1 : Ground
  IIR_BPF_Im : MATLAB Function  TreatAsAtomicUnit=on  mask{fQ=fQ, fTs=fTs, iMode=IIR2 used as BPF in SOGI}
      mask prompts: fQ "Quality factor"; fTs "Sample time [s]"; iMode "Modes of 2nd-order transfer function"
  IIR_BPF_Re1 : MATLAB Function  TreatAsAtomicUnit=on  mask{fQ=fQ, fTs=fTs, iMode=IIR2 used as BPF in SOGI}
      mask prompts: fQ "Quality factor"; fTs "Sample time [s]"; iMode "Modes of 2nd-order transfer function"
  IIR_LPF_Im : MATLAB Function  TreatAsAtomicUnit=on  mask{fQ=fQ, fTs=fTs, iMode=IIR2 used as LPF in SOGI}
      mask prompts: fQ "Quality factor"; fTs "Sample time [s]"; iMode "Modes of 2nd-order transfer function"
  IIR_LPF_Re1 : MATLAB Function  TreatAsAtomicUnit=on  mask{fQ=fQ, fTs=fTs, iMode=IIR2 used as LPF in SOGI}
      mask prompts: fQ "Quality factor"; fTs "Sample time [s]"; iMode "Modes of 2nd-order transfer function"
  Mux : Mux  Inputs=3
  Mux1 : Mux  Inputs=3
  Mux2 : Mux
  Subtract1 : Sum  Inputs=+-
  Subtract2 : Sum
  Terminator : Terminator
  RizPos : Outport
  RizNeg : Outport  Port=2
  chk : Outport  Port=3
  wires:
  [ImBP] -> Add2/2
  [ffc] -> IIR_BPF_Im/2(fn)
  Add1/1 -> Gain3/1
  [ReLP] -> Mux2/3
  [ImBP] -> Mux2/4
  Demux1/1 -> [Re]
  RIZ/1 -> [Riz]
  Ground1/1 -> Mux1/3
  [ImLP] -> Mux2/2
  Add2/1 -> Gain4/1
  [ImLP] -> Subtract1/2
  [ReLP] -> Add1/1
  [ReBP] -> Subtract2/1
  [ImBP] -> Add1/2
  Gain1/1 -> [ReNeg]
  IIR_LPF_Re1/1(y) -> [ReLP]
  [Re] -> IIR_BPF_Re1/1(u)
  [RePos] -> Mux/1
  [ReBP] -> Subtract1/1
  Mux/1 -> RizPos/1
  [ffc] -> IIR_BPF_Re1/2(fn)
  Mux1/1 -> RizNeg/1
  IIR_BPF_Im/1(y) -> [ImBP]
  [Im] -> IIR_BPF_Im/1(u)
  Demux1/3 -> Terminator/1
  IIR_BPF_Re1/1(y) -> [ReBP]
  Gain3/1 -> [ImPos]
  IIR_LPF_Im/1(y) -> [ImLP]
  [ImNeg] -> Mux1/2
  [Im] -> IIR_LPF_Im/1(u)
  [ffc] -> IIR_LPF_Im/2(fn)
  [ImLP] -> Subtract2/2
  Demux1/2 -> [Im]
  Subtract1/1 -> Gain2/1
  [Re] -> IIR_LPF_Re1/1(u)
  [ffc] -> IIR_LPF_Re1/2(fn)
  [ReBP] -> Mux2/1
  [Riz] -> Demux1/1
  Ground/1 -> Mux/3
  [ReNeg] -> Mux1/1
  Mux2/1 -> chk/1
  Gain4/1 -> [ImNeg]
  Subtract2/1 -> Gain1/1
  Gain2/1 -> [RePos]
  [ReLP] -> Add2/1
  ffc/1 -> [ffc]
  [ImPos] -> Mux/2

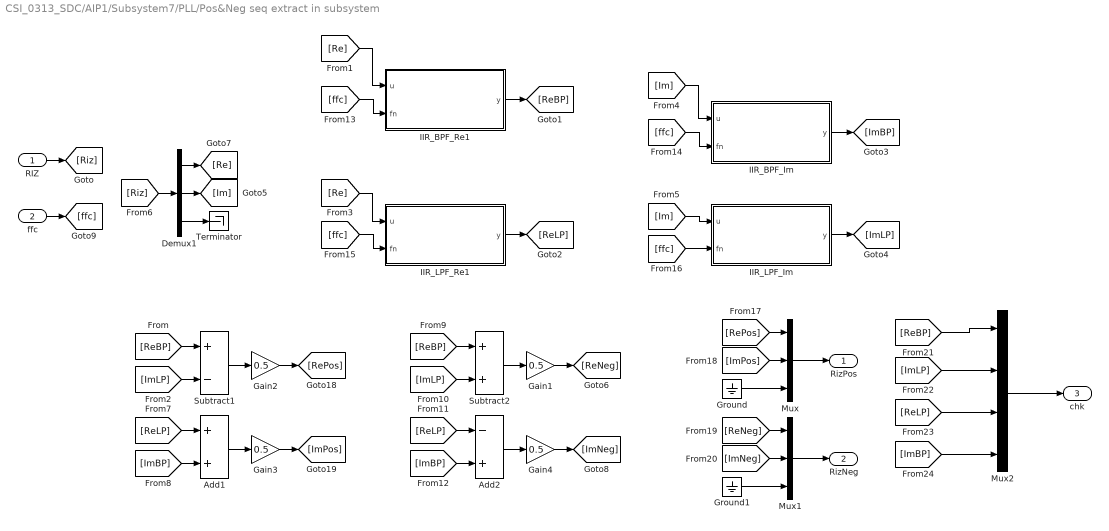
== system CSI_0313_SDC/AIP1/Subsystem7/PLL/Pos&Neg seq extract in subsystem  ==
  RIZ : Inport
  ffc : Inport  Port=2
  Add1 : Sum
  Add2 : Sum  Inputs=-+
  Demux1 : Demux  Outputs=3
  Gain{1..4} (4 alike) : Gain  Gain=0.5
  Ground : Ground
  Ground1 : Ground
  IIR_BPF_Im : MATLAB Function  TreatAsAtomicUnit=on  mask{fQ=fQ, fTs=fTs, iMode=IIR2 used as BPF in SOGI}
      mask prompts: fQ "Quality factor"; fTs "Sample time [s]"; iMode "Modes of 2nd-order transfer function"
  IIR_BPF_Re1 : MATLAB Function  TreatAsAtomicUnit=on  mask{fQ=fQ, fTs=fTs, iMode=IIR2 used as BPF in SOGI}
      mask prompts: fQ "Quality factor"; fTs "Sample time [s]"; iMode "Modes of 2nd-order transfer function"
  IIR_LPF_Im : MATLAB Function  TreatAsAtomicUnit=on  mask{fQ=fQ, fTs=fTs, iMode=IIR2 used as LPF in SOGI}
      mask prompts: fQ "Quality factor"; fTs "Sample time [s]"; iMode "Modes of 2nd-order transfer function"
  IIR_LPF_Re1 : MATLAB Function  TreatAsAtomicUnit=on  mask{fQ=fQ, fTs=fTs, iMode=IIR2 used as LPF in SOGI}
      mask prompts: fQ "Quality factor"; fTs "Sample time [s]"; iMode "Modes of 2nd-order transfer function"
  Mux : Mux  Inputs=3
  Mux1 : Mux  Inputs=3
  Mux2 : Mux
  Subtract1 : Sum  Inputs=+-
  Subtract2 : Sum
  Terminator : Terminator
  RizPos : Outport
  RizNeg : Outport  Port=2
  chk : Outport  Port=3
  wires:
  [ImBP] -> Add2/2
  [ffc] -> IIR_BPF_Im/2(fn)
  Add1/1 -> Gain3/1
  [ReLP] -> Mux2/3
  [ImBP] -> Mux2/4
  Demux1/1 -> [Re]
  RIZ/1 -> [Riz]
  Ground1/1 -> Mux1/3
  [ImLP] -> Mux2/2
  Add2/1 -> Gain4/1
  [ImLP] -> Subtract1/2
  [ReLP] -> Add1/1
  [ReBP] -> Subtract2/1
  [ImBP] -> Add1/2
  Gain1/1 -> [ReNeg]
  IIR_LPF_Re1/1(y) -> [ReLP]
  [Re] -> IIR_BPF_Re1/1(u)
  [RePos] -> Mux/1
  [ReBP] -> Subtract1/1
  Mux/1 -> RizPos/1
  [ffc] -> IIR_BPF_Re1/2(fn)
  Mux1/1 -> RizNeg/1
  IIR_BPF_Im/1(y) -> [ImBP]
  [Im] -> IIR_BPF_Im/1(u)
  Demux1/3 -> Terminator/1
  IIR_BPF_Re1/1(y) -> [ReBP]
  Gain3/1 -> [ImPos]
  IIR_LPF_Im/1(y) -> [ImLP]
  [ImNeg] -> Mux1/2
  [Im] -> IIR_LPF_Im/1(u)
  [ffc] -> IIR_LPF_Im/2(fn)
  [ImLP] -> Subtract2/2
  Demux1/2 -> [Im]
  Subtract1/1 -> Gain2/1
  [Re] -> IIR_LPF_Re1/1(u)
  [ffc] -> IIR_LPF_Re1/2(fn)
  [ReBP] -> Mux2/1
  [Riz] -> Demux1/1
  Ground/1 -> Mux/3
  [ReNeg] -> Mux1/1
  Mux2/1 -> chk/1
  Gain4/1 -> [ImNeg]
  Subtract2/1 -> Gain1/1
  Gain2/1 -> [RePos]
  [ReLP] -> Add2/1
  ffc/1 -> [ffc]
  [ImPos] -> Mux/2

== system CSI_0313_SDC/AIP1/Subsystem7/Pos Compensation/Signal Builder ==
  Demux : Demux  Tag=STV Demux  Outputs=1
  FromWs : FromWorkspace  Tag=STV FromWs  VariableName=tuvar
      SigBuilderData=|
      | common.afterFinalStr = 'Extrapolate'
      | common.sampleTime = '-1'
      | dataSet.timeRange = [0 10]
      | dataSet.name = 'Group 1'
      | sbobj.Groups.Name = 'Group 1'
      | sbobj.Groups.Signals.Name = 'Signal 1'
      | sbobj.Groups.Signals.XData = [0 1 1 2 2 3 3 10]
      | sbobj.Groups.Signals.YData = [610 610 630 630 650 650 700 700]
  Signal 1 : Outport  Tag=STV Outport  VectorParamsAs1DForOutWhenUnconnected=off
  wires:
  Demux/1 -> Signal 1/1
  FromWs/1 -> Demux/1

== system CSI_0313_SDC/AIP1/Subsystem7/Pos Compensation1/Signal Builder ==
  Demux : Demux  Tag=STV Demux  Outputs=1
  FromWs : FromWorkspace  Tag=STV FromWs  VariableName=tuvar
      SigBuilderData=|
      | common.afterFinalStr = 'Extrapolate'
      | common.sampleTime = '-1'
      | dataSet.timeRange = [0 10]
      | dataSet.name = 'Group 1'
      | sbobj.Groups.Name = 'Group 1'
      | sbobj.Groups.Signals.Name = 'Signal 1'
      | sbobj.Groups.Signals.XData = [0 0.5 0.5 2 2 3 3 10]
      | sbobj.Groups.Signals.YData = [650 650 630 630 650 650 700 700]
  Signal 1 : Outport  Tag=STV Outport  VectorParamsAs1DForOutWhenUnconnected=off
  wires:
  FromWs/1 -> Demux/1
  Demux/1 -> Signal 1/1

== matlab function CSI_0313_SDC/AIP1/SPWM_Three Level/Voltage update timing generator1 ==
  data: Trigger input; Tupdate output; Update input
function Tupdate = fcn(Trigger,Update)
    persistent cntx Tupdate1;
    if isempty(cntx)
         if(Update == 1)
            cntx =  1;
         else
            cntx =  3;
         end
        Tupdate1 = 0;
    end
    
    if(Trigger > 0)
        cntx = cntx +1;
    else
        cntx = cntx;
    end
    
    
    if(Trigger > 0 && cntx == 2)
        Tupdate1 = Trigger;
    else
        Tupdate1 = 0;        
    end
    if(cntx == 2*Update)
        cntx = 0;
    end

    Tupdate = Tupdate1;

== matlab function CSI_0313_SDC/AIP1/Moving average2 ==
  data: yout output; uin input; trig input; iNumAvg parameter; iNumDly parameter; ubase parameter
function yout=sample(uin,trig,iNumAvg,iNumDly,ubase)

persistent uary cnt sum yavg;

iNumIn = length(uin);
iNumDly = iNumDly+1;
if isempty(cnt)  
    cnt = 0;
    uary = zeros(iNumIn,iNumAvg);
    sum = zeros(iNumIn,1);
    yavg = zeros(iNumIn,iNumDly);   
end

if(trig >0) 
    for i=1:1:iNumIn
        for j=iNumDly:-1:2
            yavg(i,j)= yavg(i,j-1);
        end
    end
    cnt = cnt +1;
    for i=1:1:iNumIn
         uary(i,cnt) = uin(i)/ubase;            
        for j=1:1:iNumAvg
        sum(i) = sum(i)+uary(i,j);
        end
    end
       for i=1:1:iNumIn
            yavg(i,1)=sum(i)/iNumAvg;
       end
        
        for i=1:1:iNumIn
            sum(i)=0;
        end
        if(cnt >= iNumAvg)
            cnt = 0;
        end
end
    yout = yavg(:,iNumDly);
end

== matlab function CSI_0313_SDC/AIP1/Subsystem4/IIR_1st1 ==
  data: u input; fc parameter; y output; fTs parameter
function y = IIR_1st(u, fc, fTs)
    % y[n] = (-(1-T)*y[n-1] + x[n] + x[n-1])/(1+T)
    % u:    Input
    % fc:   Cut-off frequency
    % fTs:  Sample time
    
    persistent t;
    
    if isempty(t)
        t = zeros(2,2);
    end
    
    T = 1/(pi*fc*fTs);            
    
%     if(Trig > 0)
        t(1,1) = u;        
        t(2,1) = (t(1,1) + t(1,2) - (1-T)*t(2,2)) / (1+T);
    
        t(1,2) = t(1,1);
        t(2,2) = t(2,1);
%     else
%         t(1,1) = t(1,1);        
%         t(2,1) = t(2,1);
%     
%         t(1,2) = t(1,2);
%         t(2,2) = t(2,2);
%     end
%     
    y = t(2,1);
end

== matlab function CSI_0313_SDC/AIP1/Subsystem7/ABC_To_RIZ1 ==
  data: ABC input; RIZ output
function RIZ = ABC_To_RIZ(ABC)
    % Clarke Transfer from ABC axis to Re-Im axis
    RIZ = [0;0;0];
    RIZ(1) = (2*ABC(1)-ABC(2)-ABC(3))/3;
    RIZ(2) = sqrt(3)*(ABC(2)-ABC(3))/3;
    RIZ(3) = (ABC(1)+ABC(2)+ABC(3))/3;
end

== matlab function CSI_0313_SDC/AIP1/Subsystem7/ABC_To_RIZ ==
  data: ABC input; RIZ output
function RIZ = ABC_To_RIZ(ABC)
    % Clarke Transfer from ABC axis to Re-Im axis
    RIZ = [0;0;0];
    RIZ(1) = (2*ABC(1)-ABC(2)-ABC(3))/3;
    RIZ(2) = sqrt(3)*(ABC(2)-ABC(3))/3;
    RIZ(3) = (ABC(1)+ABC(2)+ABC(3))/3;
end

== matlab function CSI_0313_SDC/AIP1/Subsystem7/Current Limitation pu Standard/ABC_To_RIZ ==
  data: ABC input; RIZ output
function RIZ = ABC_To_RIZ(ABC)
    % Clarke Transfer from ABC axis to Re-Im axis
    RIZ = [0;0;0];
    RIZ(1) = (2*ABC(1)-ABC(2)-ABC(3))/3;
    RIZ(2) = sqrt(3)*(ABC(2)-ABC(3))/3;
    RIZ(3) = (ABC(1)+ABC(2)+ABC(3))/3;
end

== matlab function CSI_0313_SDC/AIP1/Subsystem7/Current Limitation pu Standard/IIR_1st ==
  data: u input; fc parameter; y output; fTs parameter
function y = IIR_1st(u, fc, fTs)
    % y[n] = (-(1-T)*y[n-1] + x[n] + x[n-1])/(1+T)
    % u:    Input
    % fc:   Cut-off frequency
    % fTs:  Sample time
    
    persistent t;
    
    if isempty(t)
        t = zeros(2,2);
    end
    
    T = 1/(pi*fc*fTs);            
%     if(Trig > 0)
        t(1,1) = u;        
        t(2,1) = (t(1,1) + t(1,2) - (1-T)*t(2,2)) / (1+T);
    
        t(1,2) = t(1,1);
        t(2,2) = t(2,1);
%     else
%         t(1,1) = t(1,1);        
%         t(2,1) = t(2,1);
%     
%         t(1,2) = t(1,2);
%         t(2,2) = t(2,2);
%     end
    y = t(2,1);
end

== matlab function CSI_0313_SDC/AIP1/Subsystem4/IIR_1st2 ==
  data: u input; fc parameter; y output; fTs parameter
function y = IIR_1st(u, fc, fTs)
    % y[n] = (-(1-T)*y[n-1] + x[n] + x[n-1])/(1+T)
    % u:    Input
    % fc:   Cut-off frequency
    % fTs:  Sample time
    
    persistent t;
    
    if isempty(t)
        t = zeros(2,2);
    end
    
    T = 1/(pi*fc*fTs);            
    
%     if(Trig > 0)
        t(1,1) = u;        
        t(2,1) = (t(1,1) + t(1,2) - (1-T)*t(2,2)) / (1+T);
    
        t(1,2) = t(1,1);
        t(2,2) = t(2,1);
%     else
%         t(1,1) = t(1,1);        
%         t(2,1) = t(2,1);
%     
%         t(1,2) = t(1,2);
%         t(2,2) = t(2,2);
%     end
%     
    y = t(2,1);
end

== matlab function CSI_0313_SDC/AIP1/Subsystem7/Current Limitation pu Standard/IIR_1st1 ==
  data: u input; fc parameter; y output; fTs parameter
function y = IIR_1st(u, fc, fTs)
    % y[n] = (-(1-T)*y[n-1] + x[n] + x[n-1])/(1+T)
    % u:    Input
    % fc:   Cut-off frequency
    % fTs:  Sample time
    
    persistent t;
    
    if isempty(t)
        t = zeros(2,2);
    end
    
    T = 1/(pi*fc*fTs);            
    
%     if(Trig > 0)
        t(1,1) = u;        
        t(2,1) = (t(1,1) + t(1,2) - (1-T)*t(2,2)) / (1+T);
    
        t(1,2) = t(1,1);
        t(2,2) = t(2,1);
%     else
%         t(1,1) = t(1,1);        
%         t(2,1) = t(2,1);
%     
%         t(1,2) = t(1,2);
%         t(2,2) = t(2,2);
%     end
%     
    y = t(2,1);
end

== matlab function CSI_0313_SDC/AIP1/Subsystem7/Current Limitation pu Standard/IIR_1st2 ==
  data: u input; fc parameter; y output; fTs parameter
function y = IIR_1st(u, fc, fTs)
    % y[n] = (-(1-T)*y[n-1] + x[n] + x[n-1])/(1+T)
    % u:    Input
    % fc:   Cut-off frequency
    % fTs:  Sample time
    
    persistent t;
    
    if isempty(t)
        t = zeros(2,2);
    end
    
    T = 1/(pi*fc*fTs);            
    
%     if(Trig > 0)
        t(1,1) = u;        
        t(2,1) = (t(1,1) + t(1,2) - (1-T)*t(2,2)) / (1+T);
    
        t(1,2) = t(1,1);
        t(2,2) = t(2,1);
%     else
%         t(1,1) = t(1,1);        
%         t(2,1) = t(2,1);
%     
%         t(1,2) = t(1,2);
%         t(2,2) = t(2,2);
%     end
    
    y = t(2,1);
end

== matlab function CSI_0313_SDC/AIP1/Subsystem7/Current Limitation pu Standard/PI Ctrl1 ==
  data: err input; y output; fKI parameter; fMinLmt parameter; fTs parameter; fMaxLmt parameter; fKP parameter
function y = PICtrl(err, fKI, fMinLmt, fTs, fMaxLmt, fKP)
    % y[n] = y[n-1] + KP*(x[n]-x[n-1]) + (KP*KI*TS*0.5)*(x[n]+x[n-1])
    % err:  error input
    % fKP:   Proportional gain
    % fKI:   Integral Coefficient
    % fMinLmt: Minimum limitation
    % fMaxLmt: Maximum limitation
    % fTs:  Sampling time
    
    % t(1,2) stores x[n],x[n-1]; t(2,2) stores y[n],y[n-1]
    persistent t;      
    if isempty(t)           % Initialization
        t = zeros(2,2);
    end
    
%     if(Trig > 0)
        t(1,1) = err;
        t(2,1) = t(2,2) + fKP*(t(1,1)-t(1,2)) + fKP*fKI*0.5*(t(1,1)+t(1,2))*fTs;   
    
        if (t(2,1) < fMinLmt)
            t(2,1) = fMinLmt;
        elseif (t(2,1) > fMaxLmt)
            t(2,1) = fMaxLmt;
        end
    
        t(1,2) = t(1,1);
        t(2,2) = t(2,1);
%     else
%         t(1,1) = t(1,1);
%         t(2,1) = t(2,1);      
%         t(1,2) = t(1,2);
%         t(2,2) = t(2,2);
%     end
    y = t(2,1);
end

== matlab function CSI_0313_SDC/AIP1/Subsystem7/PR CSI Loop/PR Ctrl ==
  data: err input; y output; ffc input; fP parameter; fQ parameter; fTs parameter
function y = PRCtrl(err, ffc, fP, fQ, fTs)
    % PR regulation with variant frequency input
    % y[n] = (fa1*x[n]+fa2*x[n-1]+fa3*x[n-2]-fb2*y[n-1]-fb3*y[n-2])/fb1
    % err:  error input
    % ffc:  Natural frequency
    % fP:   Proportional gain
    % fQ:   Quality factor
    % fTs:  Sampling time
    
    % t(1,3) stores x[n],x[n-1],x[n-2]; t(2,3) stores y[n],y[n-1],y[n-2]
    persistent t;      
    if isempty(t)           % Initialization
        t = zeros(2,3);
    end

    fwc = 2*pi*ffc;
    fw0 = fwc/fQ;
    
    fT1 = 2*fw0*fTs;            
    fT2 = (fwc*fTs)^2;  

    fa1 = (4+fT1+fT2)*fP;
    fa2 = (2*fT2-8)*fP;
    fa3 = (4-fT1+fT2)*fP;
    fb1 = 4+fT2;
    fb2 = 2*fT2-8;
    fb3 = 4+fT2;
%     if(Trig > 0)
        t(1,1) = err;
        t(2,1) = (fa1*t(1,1)+fa2*t(1,2)+fa3*t(1,3)-fb2*t(2,2)-fb3*t(2,3))/fb1;     
        
        t(1,3) = t(1,2);
        t(1,2) = t(1,1);
 
        t(2,3) = t(2,2);
        t(2,2) = t(2,1);
%     else
%         t(1,1) = t(1,1);
%         t(2,1) = t(2,1);     
%         
%         t(1,3) = t(1,3);
%         t(1,2) = t(1,2);
%  
%         t(2,3) = t(2,3);
%         t(2,2) = t(2,2);       
%     end
    y = t(2,1);
end

== matlab function CSI_0313_SDC/AIP1/Subsystem7/PLL/ABC_To_RIZ ==
  data: ABC input size=3; RIZ output size=3
function RIZ = ABC_To_RIZ(ABC)
    % Clarke Transfer from ABC axis to Re-Im axis
    RIZ = [0;0;0];
    RIZ(1) = (2*ABC(1)-ABC(2)-ABC(3))/3;
    RIZ(2) = sqrt(3)*(ABC(2)-ABC(3))/3;
    RIZ(3) = (ABC(1)+ABC(2)+ABC(3))/3;
end

== matlab function CSI_0313_SDC/AIP1/Subsystem7/Current Limitation pu Standard/IIR_1st3 ==
  data: u input; fc parameter; y output; fTs parameter
function y = IIR_1st(u, fc, fTs)
    % y[n] = (-(1-T)*y[n-1] + x[n] + x[n-1])/(1+T)
    % u:    Input
    % fc:   Cut-off frequency
    % fTs:  Sample time
    
    persistent t;
    
    if isempty(t)
        t = zeros(2,2);
    end
    
    T = 1/(pi*fc*fTs);            
    
%     if(Trig > 0)
        t(1,1) = u;        
        t(2,1) = (t(1,1) + t(1,2) - (1-T)*t(2,2)) / (1+T);
    
        t(1,2) = t(1,1);
        t(2,2) = t(2,1);
%     else
%         t(1,1) = t(1,1);        
%         t(2,1) = t(2,1);
%     
%         t(1,2) = t(1,2);
%         t(2,2) = t(2,2);
%     end
    
    y = t(2,1);
end

== matlab function CSI_0313_SDC/AIP1/Subsystem4/IIR_1st3 ==
  data: u input; fc parameter; y output; fTs parameter
function y = IIR_1st(u, fc, fTs)
    % y[n] = (-(1-T)*y[n-1] + x[n] + x[n-1])/(1+T)
    % u:    Input
    % fc:   Cut-off frequency
    % fTs:  Sample time
    
    persistent t;
    
    if isempty(t)
        t = zeros(2,2);
    end
    
    T = 1/(pi*fc*fTs);            
    
%     if(Trig > 0)
        t(1,1) = u;        
        t(2,1) = (t(1,1) + t(1,2) - (1-T)*t(2,2)) / (1+T);
    
        t(1,2) = t(1,1);
        t(2,2) = t(2,1);
%     else
%         t(1,1) = t(1,1);        
%         t(2,1) = t(2,1);
%     
%         t(1,2) = t(1,2);
%         t(2,2) = t(2,2);
%     end
%     
    y = t(2,1);
end

== matlab function CSI_0313_SDC/AIP1/Subsystem7/Pos&Neg seq extract in subsystem /IIR_BPF_Im ==
  data: u input; fn input; fQ parameter; y output; fTs parameter; iMode parameter
function y =IIR_2rd(u, fn, fQ, fTs, iMode)
    % Second order transfer function used for LPF and BPF
    % y[n] = (fa1*x[n]+fa2*x[n-1]+fa3*x[n-2]-fb2*y[n-1]-fb3*y[n-2])/fb1
    % u:  error input
    % fn:  Natural frequency
    % fQ:   Quality factor
    % fTs:  Sampling time
    % iMode: Mode Selection
    % iMode=1 used as generalized 2nd-order LPF, LPF(s)=wn^2/(s^2+wn/Q*s+wn^2)
    % iMode=2 used as 2nd-order LPF in SOGI, SOGI_LPF(s)=(wn^2/Q)/(s^2+wn/Q*s+wn^2)
    % iMode=3 used as 2nd-order BPF in SOGI, SOGI_BPF(s)=(wn*s/Q)/(s^2+wn/Q*s+wn^2)
    
    persistent t;
    
    if isempty(t)
        t = zeros(2,3);
    end
    
    wn = 2*pi*fn;
    wc = wn/fQ;

    fT1 = wc*wn*fTs*fTs; 
    fT2 = 2*wc*fTs;
    fT3 = (wn*fTs)^2;
    
    fb1 = fT3+fT2+4;
    fb2 = 2*fT3-8;
    fb3 = fT3-fT2+4;
    
    if (iMode ==1)
        fa1 = fT3;
        fa2 = 2*fT3;
        fa3 = fT3;
    elseif (iMode ==2)
        fa1 = fT1;
        fa2 = 2*fT1;
        fa3 = fT1;
    else
        fa1 = fT2;
        fa2 = 0;
        fa3 = -fT2;
    end
        
%     if(Trigs > 0)
        t(1,1) = u;        
        t(2,1) = (fa1*t(1,1)+fa2*t(1,2)+fa3*t(1,3)-fb2*t(2,2)-fb3*t(2,3))/fb1;
    
        t(1,3) = t(1,2);
        t(1,2) = t(1,1);
        
        t(2,3) = t(2,2);
        t(2,2) = t(2,1);
%     else
%         t(1,1) = t(1,1);        
%         t(2,1) = t(2,1);
%     
%         t(1,3) = t(1,3);
%         t(1,2) = t(1,2);
%         
%         t(2,3) = t(2,3);
%         t(2,2) = t(2,2);
%     end
    
    y = t(2,1);    
end
